simulink model "Z_3Dctrl_updated_but_still_xiaodong"  (R2023a)
settings: Solver=ode1  StartTime=0.0  StopTime=inf  FixedStep=0.001  RelTol=1e-3  EnableMultiTasking=on
PostLoadFcn:
  | , if any(exist('dsrtsu_mdlpostloadfcn', 'file') ~= 0), dsrtsu_mdlpostloadfcn('Execute', bdroot); end,
InitFcn:
  | , if any(exist('rtifpga_mdlclblib', 'file') ~= 0), rtifpga_mdlclblib('Init', bdroot); end,
  | [b,a] = butter(6,0.6)
  | z0_default = 0.080001
  | fatness_default = 1
  | offset_default = 0
  | scale_default = 0
  | tic
model workspace (MAT data in the model file):
  Iters = 5
  N_coils = 6
  fatness_default = 1
  running = 0
  z0_default = 0.080001
undefined symbols (not defined in the file): a, b, DiscIntNeverNeededParam
libraries: dspstat3 x7, simulink x4, commfilt2 x3, rti2004lib x3, rtilibm x1
(part 2 of 2)

== system Z_3Dctrl_updated_but_still_xiaodong/RTI Data/RTI Data Store/RTI Data Store/RTI Data Store ==
  RTI Data Store : Subsystem  mask(RTI_DATA_STORE){}
      mask help:
      | RTI Data Store Block. This block is used by RTI to store internal model dependent data. Deleting this block will result in data loss.
      |
      | NEVER DELETE, COPY, OR MODIFY THIS BLOCK!
      mask Help:
      | RTI Data Store Block. This block is used by RTI to store internal model dependent data. Deleting this block will result in data loss.
      | 
      | NEVER DELETE, COPY, OR MODIFY THIS BLOCK!
      mask Display: text(0.5, 0.5, ' ', 'HorizontalAlignment', 'center');

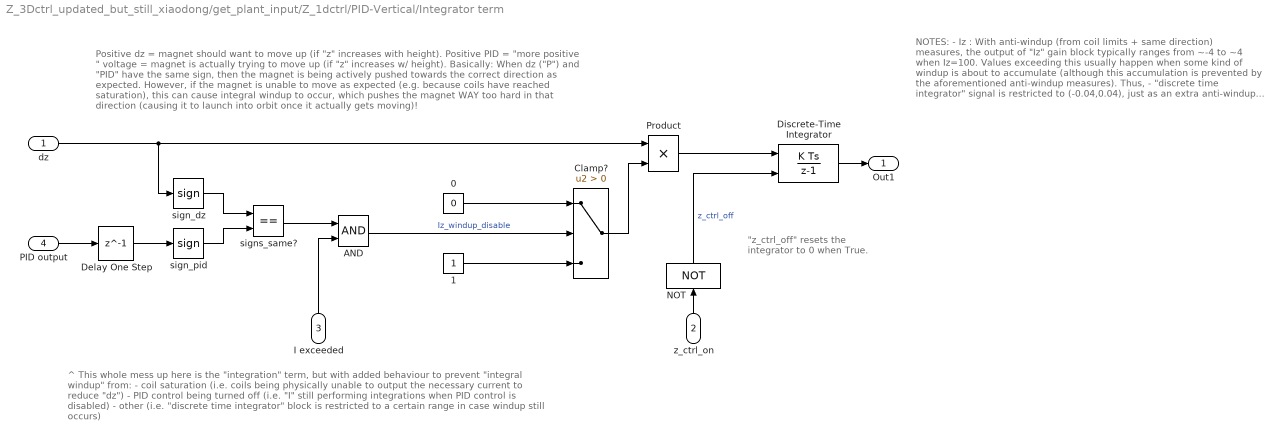
== system Z_3Dctrl_updated_but_still_xiaodong/get_plant_input/Z_1dctrl/PID-Vertical/Integrator term ==
  note: "z_ctrl_off" resets the integrator to 0 when True.
  note: Positive dz = magnet should want to move up (if "z" increases with height).
      | Positive PID = "more positive " voltage = magnet is actually trying to move up (if "z" increases w/ height).
      |
      | Basically: When dz ("P") and "PID" have the same sign, then the magnet is being actively pushed towards the correct direction as expected. However, if the magnet is unable to move as expected (e.g. because coils have reached saturation), this can cause integral windup to occur, which pushes the magnet WAY too hard in that direction (causing it to launch into orbit once it actually gets moving)!
  note: NOTES:
      | - Iz : With anti-windup (from coil limits + same direction) measures, the output of "Iz" gain block typically ranges from ~-4 to ~4 when Iz=100. Values exceeding this usually happen when some kind of windup is about to accumulate (although this accumulation is prevented by the aforementioned anti-windup measures).
      | Thus,
      | - "discrete time integrator" signal is restricted to (-0.04,0.04), just as an extra anti-windup measure.
      | - Also, the integral resets while z-control is disabled.
  note: ^ This whole mess up here is the "integration" term, but with added behaviour to prevent "integral windup" from:
      | - coil saturation (i.e. coils being physically unable to output the necessary current to reduce "dz")
      | - PID control being turned off (i.e. "I" still performing integrations when PID control is disabled)
      | - other (i.e. "discrete time integrator" block is restricted to a certain range in case windup still occurs)
  dz : Inport
  z_ctrl_on : Inport  Port=2
  I exceeded : Inport  Port=3
  PID output : Inport  Port=4
  0 : Constant  Value=0
  1 : Constant
  AND : Logic  AllPortsSameDT=off  OutDataTypeStr=boolean
  Clamp? : Switch  Criteria=u2 > Threshold  SaturateOnIntegerOverflow=off  InputSameDT=off
  Delay One Step : Delay  DelayLength=1
  Discrete-Time Integrator : DiscreteIntegrator  ExternalReset=sampled level  SampleTime=-1  LimitOutput=on  UpperSaturationLimit=0.04  LowerSaturationLimit=-0.04  ICPrevOutput=DiscIntNeverNeededParam  ICPrevScaledInput=DiscIntNeverNeededParam
  NOT : Logic  Operator=NOT  AllPortsSameDT=off  OutDataTypeStr=boolean
  Product : Product
  sign_dz : Signum
  sign_pid : Signum
  signs_same? : RelationalOperator  Operator===  OutDataTypeStr=boolean  RndMeth=Simplest  InputSameDT=off
  Out1 : Outport
  wires:
  sign_dz/1 -> signs_same?/1
  AND/1 -> Clamp?/2  "Iz_windup_disable"
  signs_same?/1 -> AND/1
  sign_pid/1 -> signs_same?/2
  1/1 -> Clamp?/3
  NOT/1 -> Discrete-Time Integrator/2  "z_ctrl_off"
  0/1 -> Clamp?/1
  Product/1 -> Discrete-Time Integrator/1
  dz/1 -> sign_dz/1, Product/1
  Clamp?/1 -> Product/2
  PID output/1 -> Delay One Step/1
  Discrete-Time Integrator/1 -> Out1/1
  z_ctrl_on/1 -> NOT/1
  I exceeded/1 -> AND/2
  Delay One Step/1 -> sign_pid/1

== system Z_3Dctrl_updated_but_still_xiaodong/get_plant_input/Z_1dctrl/PID-Vertical/PID Gain scheduler ==
  Zd : Inport
  dz : Inport  Port=2
  Dz : Constant  Value=nan
  Iz : Constant  Value=nan
  PID selector : MATLAB Function  TreatAsAtomicUnit=on
  Pz : Constant  Value=nan
  "[Pz, Iz, Dz_outer, Dz_inner, z] array" : Constant  Value=[400 2000 3200 3200 0.002; 310 350 5500 4000 0.005]
  dz_inner_threshold_mm : Constant  Value=0.1
  dz_outer_threshold_mm : Constant  Value=0.25
  PID_gains : Outport
  wires:
  Zd/1 -> PID selector/1(Zd)
  Iz/1 -> PID selector/7(I_override)
  Dz/1 -> PID selector/8(D_override)
  dz/1 -> PID selector/2(dz)
  dz_outer_threshold_mm/1 -> PID selector/5(dz_outer_threshold)
  "[Pz, Iz, Dz_outer, Dz_inner, z] array"/1 -> PID selector/3(PIDDz_save)
  Pz/1 -> PID selector/6(P_override)
  dz_inner_threshold_mm/1 -> PID selector/4(dz_inner_threshold)
  PID selector/1(PID_out) -> PID_gains/1

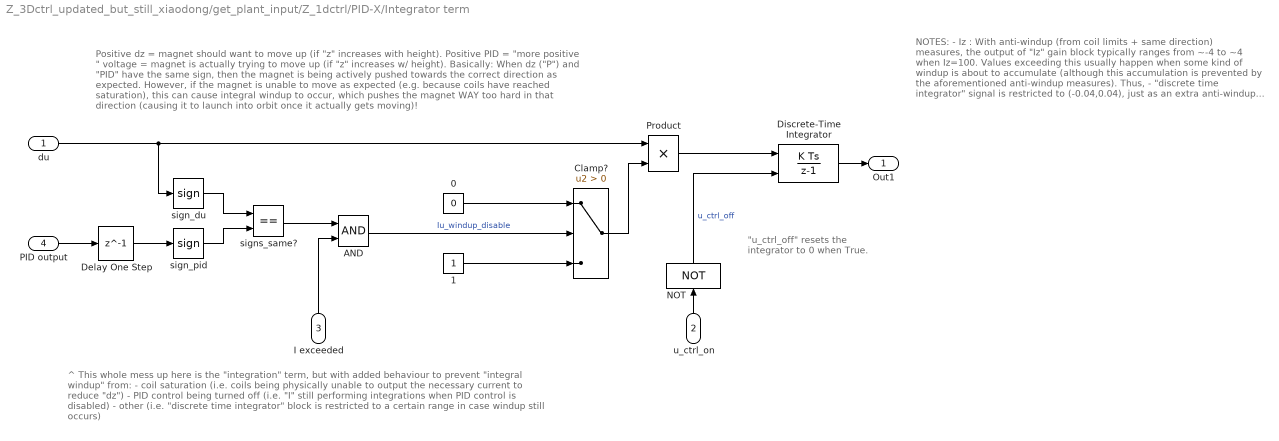
== system Z_3Dctrl_updated_but_still_xiaodong/get_plant_input/Z_1dctrl/PID-X/Integrator term ==
  note: "u_ctrl_off" resets the integrator to 0 when True.
  note: Positive dz = magnet should want to move up (if "z" increases with height).
      | Positive PID = "more positive " voltage = magnet is actually trying to move up (if "z" increases w/ height).
      |
      | Basically: When dz ("P") and "PID" have the same sign, then the magnet is being actively pushed towards the correct direction as expected. However, if the magnet is unable to move as expected (e.g. because coils have reached saturation), this can cause integral windup to occur, which pushes the magnet WAY too hard in that direction (causing it to launch into orbit once it actually gets moving)!
  note: NOTES:
      | - Iz : With anti-windup (from coil limits + same direction) measures, the output of "Iz" gain block typically ranges from ~-4 to ~4 when Iz=100. Values exceeding this usually happen when some kind of windup is about to accumulate (although this accumulation is prevented by the aforementioned anti-windup measures).
      | Thus,
      | - "discrete time integrator" signal is restricted to (-0.04,0.04), just as an extra anti-windup measure.
      | - Also, the integral resets while z-control is disabled.
  note: ^ This whole mess up here is the "integration" term, but with added behaviour to prevent "integral windup" from:
      | - coil saturation (i.e. coils being physically unable to output the necessary current to reduce "dz")
      | - PID control being turned off (i.e. "I" still performing integrations when PID control is disabled)
      | - other (i.e. "discrete time integrator" block is restricted to a certain range in case windup still occurs)
  du : Inport
  u_ctrl_on : Inport  Port=2
  I exceeded : Inport  Port=3
  PID output : Inport  Port=4
  0 : Constant  Value=0
  1 : Constant
  AND : Logic  AllPortsSameDT=off  OutDataTypeStr=boolean
  Clamp? : Switch  Criteria=u2 > Threshold  SaturateOnIntegerOverflow=off  InputSameDT=off
  Delay One Step : Delay  DelayLength=1
  Discrete-Time Integrator : DiscreteIntegrator  ExternalReset=sampled level  SampleTime=-1  LimitOutput=on  UpperSaturationLimit=0.04  LowerSaturationLimit=-0.04  ICPrevOutput=DiscIntNeverNeededParam  ICPrevScaledInput=DiscIntNeverNeededParam
  NOT : Logic  Operator=NOT  AllPortsSameDT=off  OutDataTypeStr=boolean
  Product : Product
  sign_du : Signum
  sign_pid : Signum
  signs_same? : RelationalOperator  Operator===  OutDataTypeStr=boolean  RndMeth=Simplest  InputSameDT=off
  Out1 : Outport
  wires:
  sign_du/1 -> signs_same?/1
  AND/1 -> Clamp?/2  "Iu_windup_disable"
  signs_same?/1 -> AND/1
  sign_pid/1 -> signs_same?/2
  1/1 -> Clamp?/3
  NOT/1 -> Discrete-Time Integrator/2  "u_ctrl_off"
  0/1 -> Clamp?/1
  Product/1 -> Discrete-Time Integrator/1
  du/1 -> sign_du/1, Product/1
  Clamp?/1 -> Product/2
  PID output/1 -> Delay One Step/1
  Discrete-Time Integrator/1 -> Out1/1
  u_ctrl_on/1 -> NOT/1
  I exceeded/1 -> AND/2
  Delay One Step/1 -> sign_pid/1

== system Z_3Dctrl_updated_but_still_xiaodong/get_plant_input/Z_1dctrl/PID-X/PID Gain scheduler ==
  Ud : Inport
  du : Inport  Port=2
  Du : Constant  Value=0
  Iu : Constant  Value=0
  Mux : Mux  Inputs=3
  PID selector : MATLAB Function  Commented=on  TreatAsAtomicUnit=on
  Pu : Constant  Value=50
  Terminator : Terminator  Commented=on
  Terminator1 : Terminator
  Terminator2 : Terminator
  "[Pu, Iu, Du_outer, Du_inner, z] array" : Constant  Commented=on  Value=[400 2000 3200 3200 0.002; 310 350 5500 4000 0.005]
  du_inner_threshold_mm : Constant  Commented=on  Value=0.1
  du_outer_threshold_mm : Constant  Commented=on  Value=0.25
  PID_gains : Outport
  wires:
  Ud/1 -> Terminator1/1
  Iu/1 -> Mux/2
  Du/1 -> Mux/3
  du/1 -> Terminator2/1
  du_outer_threshold_mm/1 -> PID selector/5(du_outer_threshold)
  "[Pu, Iu, Du_outer, Du_inner, z] array"/1 -> PID selector/3(PIDDu_save)
  Pu/1 -> Mux/1
  du_inner_threshold_mm/1 -> PID selector/4(du_inner_threshold)
  PID selector/1(PID_out) -> Terminator/1
  Mux/1 -> PID_gains/1

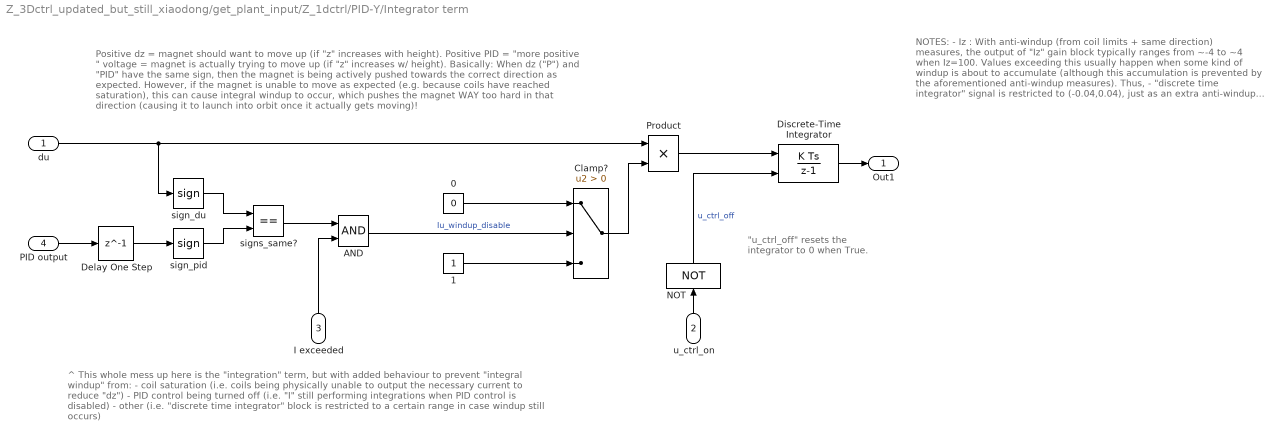
== system Z_3Dctrl_updated_but_still_xiaodong/get_plant_input/Z_1dctrl/PID-Y/Integrator term ==
  note: "u_ctrl_off" resets the integrator to 0 when True.
  note: Positive dz = magnet should want to move up (if "z" increases with height).
      | Positive PID = "more positive " voltage = magnet is actually trying to move up (if "z" increases w/ height).
      |
      | Basically: When dz ("P") and "PID" have the same sign, then the magnet is being actively pushed towards the correct direction as expected. However, if the magnet is unable to move as expected (e.g. because coils have reached saturation), this can cause integral windup to occur, which pushes the magnet WAY too hard in that direction (causing it to launch into orbit once it actually gets moving)!
  note: NOTES:
      | - Iz : With anti-windup (from coil limits + same direction) measures, the output of "Iz" gain block typically ranges from ~-4 to ~4 when Iz=100. Values exceeding this usually happen when some kind of windup is about to accumulate (although this accumulation is prevented by the aforementioned anti-windup measures).
      | Thus,
      | - "discrete time integrator" signal is restricted to (-0.04,0.04), just as an extra anti-windup measure.
      | - Also, the integral resets while z-control is disabled.
  note: ^ This whole mess up here is the "integration" term, but with added behaviour to prevent "integral windup" from:
      | - coil saturation (i.e. coils being physically unable to output the necessary current to reduce "dz")
      | - PID control being turned off (i.e. "I" still performing integrations when PID control is disabled)
      | - other (i.e. "discrete time integrator" block is restricted to a certain range in case windup still occurs)
  du : Inport
  u_ctrl_on : Inport  Port=2
  I exceeded : Inport  Port=3
  PID output : Inport  Port=4
  0 : Constant  Value=0
  1 : Constant
  AND : Logic  AllPortsSameDT=off  OutDataTypeStr=boolean
  Clamp? : Switch  Criteria=u2 > Threshold  SaturateOnIntegerOverflow=off  InputSameDT=off
  Delay One Step : Delay  DelayLength=1
  Discrete-Time Integrator : DiscreteIntegrator  ExternalReset=sampled level  SampleTime=-1  LimitOutput=on  UpperSaturationLimit=0.04  LowerSaturationLimit=-0.04  ICPrevOutput=DiscIntNeverNeededParam  ICPrevScaledInput=DiscIntNeverNeededParam
  NOT : Logic  Operator=NOT  AllPortsSameDT=off  OutDataTypeStr=boolean
  Product : Product
  sign_du : Signum
  sign_pid : Signum
  signs_same? : RelationalOperator  Operator===  OutDataTypeStr=boolean  RndMeth=Simplest  InputSameDT=off
  Out1 : Outport
  wires:
  sign_du/1 -> signs_same?/1
  AND/1 -> Clamp?/2  "Iu_windup_disable"
  signs_same?/1 -> AND/1
  sign_pid/1 -> signs_same?/2
  1/1 -> Clamp?/3
  NOT/1 -> Discrete-Time Integrator/2  "u_ctrl_off"
  0/1 -> Clamp?/1
  Product/1 -> Discrete-Time Integrator/1
  du/1 -> sign_du/1, Product/1
  Clamp?/1 -> Product/2
  PID output/1 -> Delay One Step/1
  Discrete-Time Integrator/1 -> Out1/1
  u_ctrl_on/1 -> NOT/1
  I exceeded/1 -> AND/2
  Delay One Step/1 -> sign_pid/1

== system Z_3Dctrl_updated_but_still_xiaodong/get_plant_input/Z_1dctrl/PID-Y/PID Gain scheduler ==
  Ud : Inport
  du : Inport  Port=2
  Du : Constant  Value=0
  Iu : Constant  Value=0
  Mux : Mux  Inputs=3
  PID selector : MATLAB Function  Commented=on  TreatAsAtomicUnit=on
  Pu : Constant  Value=50
  Terminator : Terminator  Commented=on
  Terminator1 : Terminator
  Terminator2 : Terminator
  "[Pu, Iu, Du_outer, Du_inner, z] array" : Constant  Commented=on  Value=[400 2000 3200 3200 0.002; 310 350 5500 4000 0.005]
  du_inner_threshold_mm : Constant  Commented=on  Value=0.1
  du_outer_threshold_mm : Constant  Commented=on  Value=0.25
  PID_gains : Outport
  wires:
  Ud/1 -> Terminator1/1
  Iu/1 -> Mux/2, PID selector/7(I_override)
  Du/1 -> Mux/3, PID selector/8(D_override)
  du/1 -> Terminator2/1
  du_outer_threshold_mm/1 -> PID selector/5(du_outer_threshold)
  "[Pu, Iu, Du_outer, Du_inner, z] array"/1 -> PID selector/3(PIDDu_save)
  Pu/1 -> Mux/1, PID selector/6(P_override)
  du_inner_threshold_mm/1 -> PID selector/4(du_inner_threshold)
  PID selector/1(PID_out) -> Terminator/1
  Mux/1 -> PID_gains/1

== system Z_3Dctrl_updated_but_still_xiaodong/plant/Position Determination1/x filter/10ms mean ==
  note: NOTE: Sensor readings fluctuate over a peak-to-peak amplitude of about 4.5e-5 m, over a period of almost exactly 10ms.
      |
      | 08/14/23: See how it improves if I only consider the mean signal over 10ms!
  u : Inport
  ave signal : Product  Inputs=*/
  integration window (samples) : Constant  Value=10
  sum of signal over short time : commfilt2/Windowed Integrator  integperiod=10  InputProcessing=Columns as channels (frame based)  roundingMode=Floor  overflowMode=off  coeffDataTypeStr=Inherit: Same word length as input  coeffMin=[]  coeffMax=[]  coeffLastDataTypeStr=Inherit: Same word length as input  accumDataTypeStr=Inherit: Same as product output  accumLastDataTypeStr=Inherit: Same as product output  outputDataTypeStr=Inherit: Same as accumulator  outputMin=[]  outputMax=[]  outputLastDataTypeStr=Inherit: Same as accumulator
  movingmean(u) : Outport
  wires:
  sum of signal over short time/1 -> ave signal/1
  u/1 -> sum of signal over short time/1
  integration window (samples)/1 -> ave signal/2
  ave signal/1 -> movingmean(u)/1

== system Z_3Dctrl_updated_but_still_xiaodong/plant/Position Determination1/y filter/10ms mean ==
  note: NOTE: Sensor readings fluctuate over a peak-to-peak amplitude of about 4.5e-5 m, over a period of almost exactly 10ms.
      |
      | 08/14/23: See how it improves if I only consider the mean signal over 10ms!
  u : Inport
  ave signal : Product  Inputs=*/
  integration window (samples) : Constant  Value=10
  sum of signal over short time : commfilt2/Windowed Integrator  integperiod=10  InputProcessing=Columns as channels (frame based)  roundingMode=Floor  overflowMode=off  coeffDataTypeStr=Inherit: Same word length as input  coeffMin=[]  coeffMax=[]  coeffLastDataTypeStr=Inherit: Same word length as input  accumDataTypeStr=Inherit: Same as product output  accumLastDataTypeStr=Inherit: Same as product output  outputDataTypeStr=Inherit: Same as accumulator  outputMin=[]  outputMax=[]  outputLastDataTypeStr=Inherit: Same as accumulator
  movingmean(u) : Outport
  wires:
  sum of signal over short time/1 -> ave signal/1
  u/1 -> sum of signal over short time/1
  integration window (samples)/1 -> ave signal/2
  ave signal/1 -> movingmean(u)/1

== system Z_3Dctrl_updated_but_still_xiaodong/plant/Position Determination1/z filter SMOOTH/10ms mean ==
  note: NOTE: Sensor readings fluctuate over a peak-to-peak amplitude of about 4.5e-5 m, over a period of almost exactly 10ms.
      |
      | 08/14/23: See how it improves if I only consider the mean signal over 10ms!
  u : Inport
  ave signal : Product  Inputs=*/
  integration window (samples) : Constant  Value=10
  sum of signal over short time : commfilt2/Windowed Integrator  integperiod=10  InputProcessing=Columns as channels (frame based)  roundingMode=Floor  overflowMode=off  coeffDataTypeStr=Inherit: Same word length as input  coeffMin=[]  coeffMax=[]  coeffLastDataTypeStr=Inherit: Same word length as input  accumDataTypeStr=Inherit: Same as product output  accumLastDataTypeStr=Inherit: Same as product output  outputDataTypeStr=Inherit: Same as accumulator  outputMin=[]  outputMax=[]  outputLastDataTypeStr=Inherit: Same as accumulator
  movingmean(u) : Outport
  wires:
  sum of signal over short time/1 -> ave signal/1
  u/1 -> sum of signal over short time/1
  integration window (samples)/1 -> ave signal/2
  ave signal/1 -> movingmean(u)/1

== system Z_3Dctrl_updated_but_still_xiaodong/plant/output signal/output signal diagnostics/STDs ==
  H123 : Inport
  Demux : Demux  Outputs=3
  Moving Standard Deviation : dspstat3/Moving Standard Deviation  Method=Sliding window  ForgettingFactorPort=off  SpecifyWindowLength=on  WindowLength=3000  OverlapLength=2999  AllowArbitraryInputLength=off  ForgettingFactor=0.9  SimulateUsing=Code generation
  Moving Standard Deviation1 : dspstat3/Moving Standard Deviation  Method=Sliding window  ForgettingFactorPort=off  SpecifyWindowLength=on  WindowLength=3000  OverlapLength=2999  AllowArbitraryInputLength=off  ForgettingFactor=0.9  SimulateUsing=Code generation
  Moving Standard Deviation2 : dspstat3/Moving Standard Deviation  Method=Sliding window  ForgettingFactorPort=off  SpecifyWindowLength=on  WindowLength=3000  OverlapLength=2999  AllowArbitraryInputLength=off  ForgettingFactor=0.9  SimulateUsing=Code generation
  Terminator : Terminator
  Terminator1 : Terminator
  Terminator2 : Terminator
  wires:
  H123/1 -> Demux/1
  Demux/1 -> Moving Standard Deviation/1
  Demux/2 -> Moving Standard Deviation1/1
  Demux/3 -> Moving Standard Deviation2/1
  Moving Standard Deviation/1 -> Terminator/1  "std_HZ"
  Moving Standard Deviation1/1 -> Terminator1/1  "std_HII"
  Moving Standard Deviation2/1 -> Terminator2/1  "std_HIII"

== system Z_3Dctrl_updated_but_still_xiaodong/plant/output signal/output signal diagnostics/center ==
  u : Inport
  Demux : Demux  Outputs=3
  Moving Average : dspstat3/Moving Average  Method=Sliding window  ForgettingFactorPort=off  SpecifyWindowLength=on  WindowLength=3000  OverlapLength=2999  AllowArbitraryInputLength=off  ForgettingFactor=0.9  SimulateUsing=Code generation
  Moving Average1 : dspstat3/Moving Average  Method=Sliding window  ForgettingFactorPort=off  SpecifyWindowLength=on  WindowLength=3000  OverlapLength=2999  AllowArbitraryInputLength=off  ForgettingFactor=0.9  SimulateUsing=Code generation
  Moving Average2 : dspstat3/Moving Average  Method=Sliding window  ForgettingFactorPort=off  SpecifyWindowLength=on  WindowLength=3000  OverlapLength=2999  AllowArbitraryInputLength=off  ForgettingFactor=0.9  SimulateUsing=Code generation
  Mux : Mux  Inputs=3
  Sum : Sum  Inputs=|+-
  Sum1 : Sum  Inputs=|+-
  Sum2 : Sum  Inputs=|+-
  u_cen : Outport
  wires:
  u/1 -> Demux/1
  Moving Average/1 -> Sum/2
  Demux/1 -> Sum/1, Moving Average/1
  Moving Average1/1 -> Sum1/2
  Demux/2 -> Moving Average1/1, Sum1/1
  Moving Average2/1 -> Sum2/2
  Demux/3 -> Moving Average2/1, Sum2/1
  Sum1/1 -> Mux/2
  Sum/1 -> Mux/1
  Sum2/1 -> Mux/3
  Mux/1 -> u_cen/1

== system Z_3Dctrl_updated_but_still_xiaodong/RTI Data/RTI Data Store/RTI Data Store/RTI Data Store/RTI Data Store ==

== matlab function Z_3Dctrl_updated_but_still_xiaodong/Input parameters/Magnet Specs/Magnet Physical Specs ==
  data: unit_mode input; diameter input; height input; diameter_m output; height_m output; mass_g output; B_r output; mass input; magnet_remanence_t input; errorflag output
function [diameter_m,height_m,mass_g,B_r,errorflag]= mag_specs(unit_mode,diameter,height,mass,magnet_remanence_t)
% User can specify parameters for cylindrical magnets: diameter, height 
% (units: "in" or "cm" or "mm" or "m"), mass, and either remanent B-field
% (in T or G) or magnetic dipole moment (in N*m/T, aka A*m^2).
% TO IMPLEMENT: Ring magnets!

errorflag = 0;

%%% DIMENSIONS %%%
% Dimensions, in m
% NOTE: Unit modes are:
% 1 - m
% 2 - cm
% 3 - mm
% 4 - in
if unit_mode==1
    units_to_m = 1;
elseif unit_mode==2
    units_to_m = 0.01;
elseif unit_mode==3
    units_to_m = 0.001;
elseif unit_mode==4
    units_to_m = 0.0254;
else
    % (TEMP?) Assume that the user wants metres
    units_to_m = 1;
end

% Dimensions
% if isnan(diameter)
%     diameter = diameter_detect;
% end
% if isnan(diameter_detect)
%     diameter_detect = diameter;
% end
% if isnan(height)
%     height = height_detect;
% end
% if isnan(height_detect)
%     height_detect = height;
% end
diameter_m = diameter * units_to_m;
height_m = height * units_to_m;
mass_g = mass;

%%% MAG FIELD STUFF %%%
% Mag field info (Br in Gauss or T)
if magnet_remanence_t > 1000
    % Assumes a remanence field value based on the material, in Gauss.
    % For example, an N52 magnet has 14800G, and Xiaodong's now-battered
    % magnet has 12900G.
    B_r = magnet_remanence_t / 10000;
else
    % Assumes a remanence field value based on the material, in T.
    % For example, an N52 magnet has 1.48T, and Xiaodong's now-battered
    % magnet has 1.29T.
    B_r = magnet_remanence_t / 1;
end

% (!!!!) CREATE CHART FOR CONVERSION FROM Nxx FORMAT TO REMANENCE IN T

% K&J SPECS:
%     % Assumes a grade was inputted as a string-- N52, N42, etc!
%     if lower(magfield_grade_t)=="n52"
%         B_r = 1.48;
%     elseif lower(magfield_grade_t)=="n50"
%         B_r = 1.45;
%     elseif lower(magfield_grade_t)=="n48"
%         B_r = 1.42;
%     elseif lower(magfield_grade_t)=="n45"
%         B_r = 1.35;
%     elseif lower(magfield_grade_t)=="n42"
%         B_r = 1.32;
%     elseif lower(magfield_grade_t)=="n40"
%         B_r = 1.29;
%     elseif lower(magfield_grade_t)=="n35"
%         B_r = 1.21;
%     else
%         % SHOULD NEVER HAPPEN
%         B_r = 1.48;
%         errorflag = 1;
%     end
% APPLIEDMAGNETS SPECS:
%     % Assumes a grade was inputted as a string-- N52, N42, etc!
%     if lower(magfield_grade_t)=="n52"
%         B_r = 1.48;
%     elseif lower(magfield_grade_t)=="n50"
%         B_r = 1.45;
%     elseif lower(magfield_grade_t)=="n48"
%         B_r = 1.42;
%     elseif lower(magfield_grade_t)=="n45"
%         B_r = 1.38 (rarely 1.35);
%     elseif lower(magfield_grade_t)=="n42"
%         B_r = 1.32;
%     elseif lower(magfield_grade_t)=="n40"
%         B_r = 1.29;
%     else
%         % SHOULD NEVER HAPPEN
%         B_r = 1.48;
%         errorflag = 1;
%     end
% 
% 
%

== matlab function Z_3Dctrl_updated_but_still_xiaodong/get_plant_input/Z_1dctrl/PID-X/PID Gain scheduler/PID selector ==
  data: Ud input; du input; PIDDu_save input; du_inner_threshold input; du_outer_threshold input; PID_out output; P_override input; I_override input; D_override input
function PID_out = fcn(Ud,du,PIDDu_save,du_inner_threshold, du_outer_threshold, P_override,I_override,D_override)
% Interpolates for PID gains based on target Ud, using PID gains that were
% manually tuned at various target "Z" heights (with D gain being split into
% "near target height" and "far from target height" values, to allow for
% strong D contribution without risking destabilization near convergence).
% The "D" gain is then chosen between these aforementioned values based on
% how near/far the magnet is to Zd.

% Read recorded PID gains
Zq = Ud;

Ps = PIDDu_save(:,1);
Is = PIDDu_save(:,2);
Douts = PIDDu_save(:,3);
Dins = PIDDu_save(:,4);
Zs = PIDDu_save(:,5);
[~,lowest_index] = min(Zs);
[~,highest_index] = max(Zs);


% Interpolate if necessary!
if Ud <= Zs(lowest_index)
    % disp("Below 2mm!")
    P_final = Ps(lowest_index);
    I_final = Is(lowest_index);
    Dout_final = Douts(lowest_index);
    Din_final  = Dins(lowest_index);
elseif Ud >= Zs(highest_index)
    % disp("Above 5mm!")
    P_final = Ps(highest_index);
    I_final = Is(highest_index);
    Dout_final = Douts(highest_index);
    Din_final  = Dins(highest_index);
else
    % disp("Interpolate!")
    P_final     = interp1(Zs,Ps,Zq,'spline');
    I_final     = interp1(Zs,Is,Zq,'spline');
    Dout_final  = interp1(Zs,Douts,Zq,'spline');
    Din_final   = interp1(Zs,Dins,Zq,'spline');
end



% Choose between "inner" and "outer" D gains
dz_mm = du * 1000;

if abs(dz_mm) <= du_inner_threshold
    % disp("Within inner threshold")
    D_final = Din_final;
elseif abs(dz_mm) >= du_outer_threshold
    % disp("Beyond outer threshold")
    D_final = Dout_final;
else
    % disp("In between; interpolate!")
    D_final = ( Dout_final- Din_final)*(abs(dz_mm) - du_inner_threshold)/(du_outer_threshold - du_inner_threshold) +  Din_final;
end


% Apply overrides (if any)
if ~isnan(P_override)
    P_final = P_override;
end
if ~isnan(I_override)
    I_final = I_override;
end
if ~isnan(D_override)
    D_final = D_override;
end
PID_out = [P_final, I_final, D_final];

== matlab function Z_3Dctrl_updated_but_still_xiaodong/get_plant_input/Z_1dctrl/PID-Y/PID Gain scheduler/PID selector ==
  data: Ud input; du input; PIDDu_save input; du_inner_threshold input; du_outer_threshold input; PID_out output; P_override input; I_override input; D_override input
function PID_out = fcn(Ud,du,PIDDu_save,du_inner_threshold, du_outer_threshold, P_override,I_override,D_override)
% Interpolates for PID gains based on target Ud, using PID gains that were
% manually tuned at various target "Z" heights (with D gain being split into
% "near target height" and "far from target height" values, to allow for
% strong D contribution without risking destabilization near convergence).
% The "D" gain is then chosen between these aforementioned values based on
% how near/far the magnet is to Zd.

% Read recorded PID gains
Zq = Ud;

Ps = PIDDu_save(:,1);
Is = PIDDu_save(:,2);
Douts = PIDDu_save(:,3);
Dins = PIDDu_save(:,4);
Zs = PIDDu_save(:,5);
[~,lowest_index] = min(Zs);
[~,highest_index] = max(Zs);


% Interpolate if necessary!
if Ud <= Zs(lowest_index)
    % disp("Below 2mm!")
    P_final = Ps(lowest_index);
    I_final = Is(lowest_index);
    Dout_final = Douts(lowest_index);
    Din_final  = Dins(lowest_index);
elseif Ud >= Zs(highest_index)
    % disp("Above 5mm!")
    P_final = Ps(highest_index);
    I_final = Is(highest_index);
    Dout_final = Douts(highest_index);
    Din_final  = Dins(highest_index);
else
    % disp("Interpolate!")
    P_final     = interp1(Zs,Ps,Zq,'spline');
    I_final     = interp1(Zs,Is,Zq,'spline');
    Dout_final  = interp1(Zs,Douts,Zq,'spline');
    Din_final   = interp1(Zs,Dins,Zq,'spline');
end



% Choose between "inner" and "outer" D gains
dz_mm = du * 1000;

if abs(dz_mm) <= du_inner_threshold
    % disp("Within inner threshold")
    D_final = Din_final;
elseif abs(dz_mm) >= du_outer_threshold
    % disp("Beyond outer threshold")
    D_final = Dout_final;
else
    % disp("In between; interpolate!")
    D_final = ( Dout_final- Din_final)*(abs(dz_mm) - du_inner_threshold)/(du_outer_threshold - du_inner_threshold) +  Din_final;
end


% Apply overrides (if any)
if ~isnan(P_override)
    P_final = P_override;
end
if ~isnan(I_override)
    I_final = I_override;
end
if ~isnan(D_override)
    D_final = D_override;
end
PID_out = [P_final, I_final, D_final];

== matlab function Z_3Dctrl_updated_but_still_xiaodong/get_plant_input/Z_1dctrl/PID-Vertical/max(0,|dz|-threshold) ==
  data: u_threshold_mm input; u_m input; y output
function y = dz_past_threshold(u_threshold_mm, u_m)
% Input "u" is in metres.
% Input "u_threshold" is in mm.
u_mm = u_m * 1000;    
y = max(0,abs(u_mm) - u_threshold_mm);

== matlab function Z_3Dctrl_updated_but_still_xiaodong/get_plant_input/Z_1dctrl/PID-Vertical/PID Gain scheduler/PID selector ==
  data: Zd input; dz input; PIDDz_save input; dz_inner_threshold input; dz_outer_threshold input; PID_out output; P_override input; I_override input; D_override input
function PID_out = fcn(Zd,dz,PIDDz_save,dz_inner_threshold, dz_outer_threshold, P_override,I_override,D_override)
% Interpolates for PID gains based on target Zd, using PID gains that were
% manually tuned at various target heights (with D gain being split into
% "near target height" and "far from target height" values, to allow for
% strong D contribution without risking destabilization near convergence).
% The "D" gain is then chosen between these aforementioned values based on
% how near/far the magnet is to Zd.
%
% Finally, overri

% Read recorded PID gains
Zq = Zd;

Ps = PIDDz_save(:,1);
Is = PIDDz_save(:,2);
Douts = PIDDz_save(:,3);
Dins = PIDDz_save(:,4);
Zs = PIDDz_save(:,5);
[~,lowest_index] = min(Zs);
[~,highest_index] = max(Zs);


% Interpolate if necessary!
if Zd <= Zs(lowest_index)
    % disp("Below 2mm!")
    P_final = Ps(lowest_index);
    I_final = Is(lowest_index);
    Dout_final = Douts(lowest_index);
    Din_final  = Dins(lowest_index);
elseif Zd >= Zs(highest_index)
    % disp("Above 5mm!")
    P_final = Ps(highest_index);
    I_final = Is(highest_index);
    Dout_final = Douts(highest_index);
    Din_final  = Dins(highest_index);
else
    % disp("Interpolate!")
    P_final     = interp1(Zs,Ps,Zq,'spline');
    I_final     = interp1(Zs,Is,Zq,'spline');
    Dout_final  = interp1(Zs,Douts,Zq,'spline');
    Din_final   = interp1(Zs,Dins,Zq,'spline');
end



% Choose between "inner" and "outer" D gains
dz_mm = dz * 1000;

if abs(dz_mm) <= dz_inner_threshold
    % disp("Within inner threshold")
    D_final = Din_final;
elseif abs(dz_mm) >= dz_outer_threshold
    % disp("Beyond outer threshold")
    D_final = Dout_final;
else
    % disp("In between; interpolate!")
    D_final = ( Dout_final- Din_final)*(abs(dz_mm) - dz_inner_threshold)/(dz_outer_threshold - dz_inner_threshold) +  Din_final;
end


% Apply overrides (if any)
if ~isnan(P_override)
    P_final = P_override;
end
if ~isnan(I_override)
    I_final = I_override;
end
if ~isnan(D_override)
    D_final = D_override;
end
PID_out = [P_final, I_final, D_final];

== matlab function Z_3Dctrl_updated_but_still_xiaodong/plant/output signal/output signal diagnostics/butterworth ==
  data: order input; bee output; Wn input; aye output
function [bee,aye] = butterwort(order,Wn)
% order = order of lowpass Butterworth filter
% Wn = NORMALIZED cutoff frequency
%    = fc/(fs/2), where fc = cutoff frequency (Hz),
%                       fs = sample frequency (Hz) (1000 for our system)
%    = ratio between cutoff frequency and HALF of sample frequency!

% Ignore the order actually lmao
order = 2;
[bee,aye] = butter(order,Wn);

== matlab function Z_3Dctrl_updated_but_still_xiaodong/plant/Position Determination1/z filter SMOOTH/butterworth ==
  data: bee output; Wn input; aye output
function [bee,aye] = butterwort(Wn)
% order = order of lowpass Butterworth filter
% Wn = NORMALIZED cutoff frequency
%    = fc/(fs/2), where fc = cutoff frequency (Hz),
%                       fs = sample frequency (Hz) (1000 for our system)
%    = ratio between cutoff frequency and HALF of sample frequency!

% Ignore the order actually lmao
order = 6;
[bee,aye] = butter(order,Wn);
